simulink model "Lqr_clean"  (R2022a)
settings: Solver=ode3  StartTime=0.0  StopTime=inf  FixedStep=0.005  RelTol=1e-3
undefined symbols (not defined in the file): Angular, Gain, Linear
libraries: robotlib x15
settings Model: Creator=Ronak Jain  LastModifiedBy=Ronak Jain
settings OptimizationCC: EnhancedBackFolding=on  PassReuseOutputArgsAs=Individual arguments  ZeroExternalMemoryAtStartup=off  ZeroInternalMemoryAtStartup=off  MaxStackSize=64  OptimizeBlockOrder=speed  DifferentSizesBufferReuse=on  OptimizationCustomize=off  EfficientTunableParamExpr=on
settings DebuggingCC: ParameterTunabilityLossMsg=error
settings HardwareCC: ProdBitPerPointer=32  ProdBitPerSizeT=32  ProdBitPerPtrDiffT=32  ProdLargestAtomicFloat=None  ProdIntDivRoundTo=Undefined  ProdEndianess=Unspecified  ProdWordSize=32  ProdHWDeviceType=Generic->Unspecified (assume 32-bit Generic)
settings SFSimCC: MATLABDynamicMemAlloc=off
settings RTWCC: SystemTargetFile=ert.tlc  HardwareBoard=Robot Operating System (ROS)  TLCOptions="-aInlineSetEventsForThisBaseRateFcn=TLC_FALSE -aSuppressMultiTaskScheduler=TLC_FALSE  -aRateBasedStepFcn=0"  TemplateMakefile=ert_default_tmf  Toolchain=Catkin  TargetLang=C++
settings CodeAppCC: ForceParamTrailComments=on  IgnoreCustomStorageClasses=off  OperatorAnnotations=on  SimulinkDataObjDesc=on  SFDataObjDesc=on  InsertBlockDesc=on

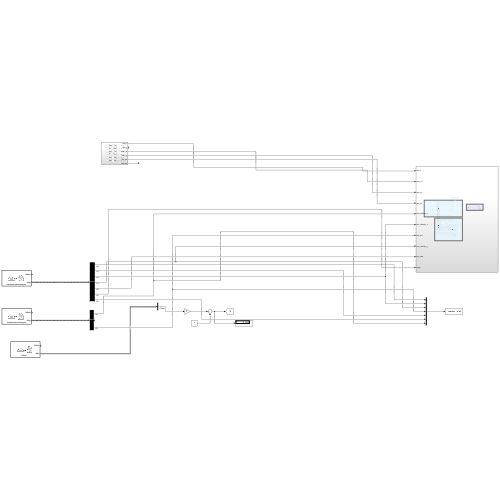
[thumbnail: Simulink's stored preview of the top-level diagram]
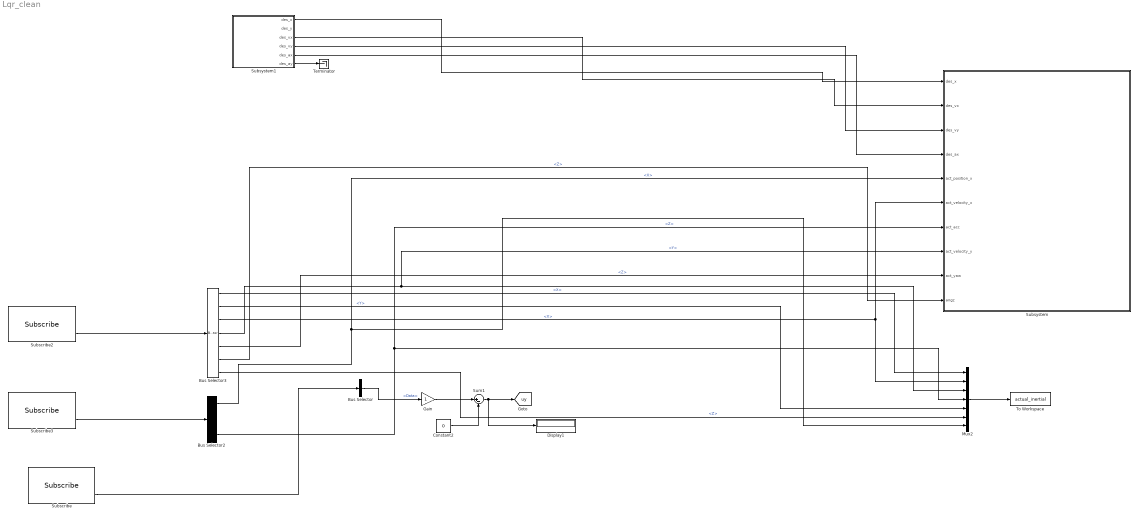
== system Lqr_clean ==
  Bus Selector : BusSelector  OutputSignals=Data
  Bus Selector2 : BusSelector  OutputSignals=LinearAcceleration.X,LinearAcceleration.Y,LinearAcceleration.Z
  Bus Selector3 : BusSelector  OutputSignals=Pose.Pose.Position.X,Pose.Pose.Position.Y,Twist.Twist.Linear.X,Twist.Twist.Linear.Y,Pose.Pose.Orientation.Z,Twist.Twist.Angular.Z,Twist.Twist.Linear.Z
  Constant2 : Constant  Value=0
  Display1 : Display
  Gain : Gain
  Mux2 : Mux  Inputs=7
  Subscribe : robotlib/Subscribe  topicSource=Select from ROS network  topic=/offset  messageType=std_msgs/Float32  SampleTime=-1  legacyBusStruct=off  messageQueueLength=1
  Subscribe2 : robotlib/Subscribe  topicSource=Select from ROS network  topic=/camera/odom/sample  messageType=nav_msgs/Odometry  SampleTime=-1  legacyBusStruct=off  messageQueueLength=1
  Subscribe3 : robotlib/Subscribe  topicSource=Select from ROS network  topic=/camera/accel/sample  messageType=sensor_msgs/Imu  SampleTime=-1  legacyBusStruct=off  messageQueueLength=1
  Subsystem : Subsystem
  Subsystem1 : Subsystem
  Sum1 : Sum  Inputs=|+-
  Terminator : Terminator
  To Workspace : ToWorkspace  VariableName=actual_inertial  SaveFormat=Timeseries  SampleTime=-1
  tag scope: uy=global
  wires:
  Subscribe/2 -> Bus Selector/1
  Bus Selector3/1 -> Mux2/1  "<X>"
  Subsystem1/6(des_ay) -> Terminator/1
  Constant2/1 -> Sum1/2
  Subsystem1/3(des_vx) -> Subsystem/2(des_vx)
  Bus Selector2/1 -> Mux2/7, Subsystem/5(act_position_x)  "<X>"
  Gain/1 -> Sum1/1
  Subscribe3/2 -> Bus Selector2/1
  Subsystem1/5(des_ax) -> Subsystem/4(des_ax)
  Sum1/1 -> Display1/1, [uy]
  Subscribe2/2 -> Bus Selector3/1
  Bus Selector3/7 -> Mux2/6  "<Z>"
  Mux2/1 -> To Workspace/1
  Bus Selector3/3 -> Subsystem/6(act_velocity_x), Mux2/2  "<X>"
  Bus Selector3/5 -> Subsystem/9(act_yaw)  "<Z>"
  Bus Selector/1 -> Gain/1  "<Data>"
  Bus Selector3/4 -> Subsystem/8(act_velocity_y), Mux2/3  "<Y>"
  Bus Selector2/3 -> Subsystem/7(act_acc), Mux2/4  "<Z>"
  Subsystem1/4(des_vy) -> Subsystem/3(des_vy)
  Bus Selector3/6 -> Subsystem/10(angz)  "<Z>"
  Bus Selector3/2 -> Mux2/5  "<Y>"
  Subsystem1/1(des_x) -> Subsystem/1(des_x)

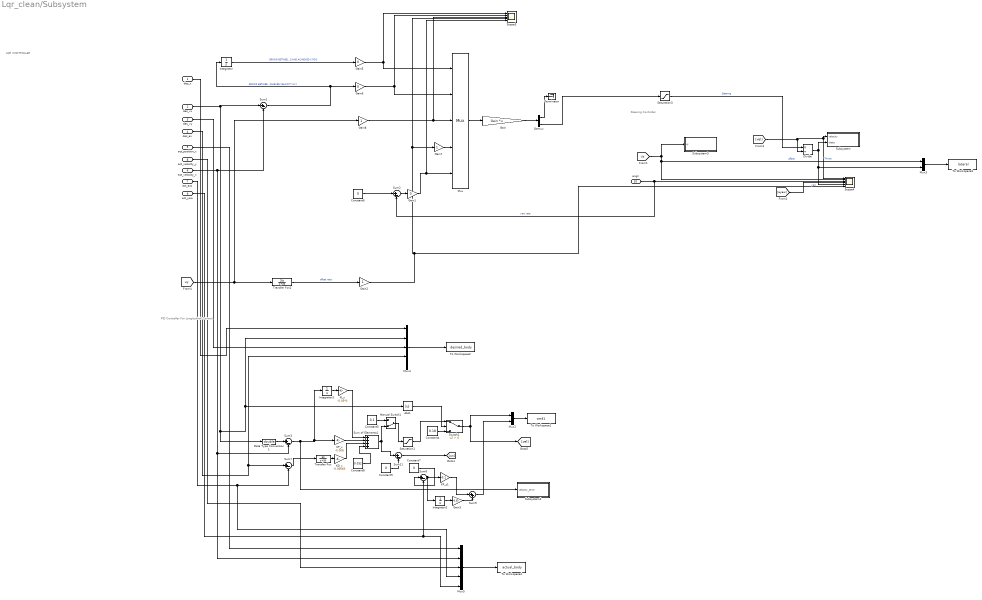
== system Lqr_clean/Subsystem ==
  note: Steering Controller
  note: LQR CONTROLLER
  note: PID Controller
      | For Longitudinal
      | Control.
  des_x : Inport
  des_vx : Inport  Port=2
  des_vy : Inport  Port=3
  des_ax : Inport  Port=4
  act_position_x : Inport  Port=5
  act_velocity_x : Inport  Port=6
  act_acc : Inport  Port=7
  act_velocity_y : Inport  Port=8
  act_yaw : Inport  Port=9
  angz : Inport  Port=10
  Abs1 : Abs  SaturateOnIntegerOverflow=off
  Constant4 : Constant  Value=0.18
  Constant5 : Constant  Value=0.1
  Constant6 : Constant  Value=0
  Constant7 : Constant  Value=0
  Constant8 : Constant  Value=0.032
  Constant9 : Constant  Value=0
  Data Type Conversion1 : DataTypeConversion  OutDataTypeStr=double  SaturateOnIntegerOverflow=off  RndMeth=Floor
  Demux : Demux  Outputs=2
  Divide : Product  Inputs=*/
  Gain : Gain  Gain=Gain  Multiplication=Matrix(K*u)
  Gain1 : Gain  Gain=0
  Gain2 : Gain
  Gain3 : Gain  Gain=-0.33
  Gain5 : Gain  Gain=0
  Gain6 : Gain  Gain=0
  Gain7 : Gain
  Gain8 : Gain
  Integrator : Integrator
  Integrator2 : Integrator
  Integrator3 : Integrator
  KD_x : Gain  Gain=-0.00083
  KI_x : Gain  Gain=-0.05*0
  KP_x : Gain  Gain=-0.008
  KP_z1 : Gain  Gain=-0.1
  Manual Switch1 : ManualSwitch  CurrentSetting=0
  Mux : Mux  Inputs=5
  Mux2 : Mux  Inputs=2
  Mux3 : Mux  Inputs=2
  Mux4 : Mux  Inputs=5
  Mux5 : Mux  Inputs=5
  Saturation1 : Saturate  LowerLimit=-0.2
  Saturation3 : Saturate  UpperLimit=0.7  LowerLimit=-0.7
  Scope3 : Scope  NumInputPorts=5
  Scope4 : Scope  NumInputPorts=6
  Subsystem : Subsystem
  Subsystem2 : Subsystem
  Subsystem3 : Subsystem
  Sum of Elements1 : Sum  Inputs=++++
  Sum{1..3,7..8,11} (6 alike) : Sum  Inputs=|+-
  Sum9 : Sum  Inputs=|++
  Switch1 : Switch  Criteria=u2 > Threshold  SaturateOnIntegerOverflow=off  InputSameDT=off
  Terminator : Terminator
  To Workspace1 : ToWorkspace  VariableName=cmd1  SaveFormat=Timeseries  SampleTime=-1
  To Workspace2 : ToWorkspace  VariableName=desired_body  SaveFormat=Timeseries  SampleTime=-1
  To Workspace3 : ToWorkspace  VariableName=lateral  SaveFormat=Timeseries  SampleTime=-1
  To Workspace4 : ToWorkspace  VariableName=actual_body  SaveFormat=Timeseries  SampleTime=-1
  Transfer Fcn : TransferFcn  Numerator=[50]  Denominator=[1 50]
  Transfer Fcn2 : TransferFcn  Numerator=[20 0]  Denominator=[1 20]
  wires:
  [uy] -> Subsystem3/1(uy), Mux3/1, Scope4/2  "offset"
  angz/1 -> Sum2/2, Scope4/3  "yaw rate"
  [ayaw] -> Scope4/4  "yaw"
  Mux3/1 -> To Workspace3/1
  [vel] -> Subsystem/1(velocity), Scope4/1, Divide/2  "Thrust"
  Sum1/1 -> Integrator/1, Gain6/1  "ERROR BETWEEN DESIRED VELOXITY IN X AND ACHIEVED VELOCITY IN X"
  Integrator/1 -> Gain5/1  "ERROR BETWEEN DESIRED X POS AND ACHIEVED X POS"
  [uy] -> Transfer Fcn2/1, Gain8/1
  Transfer Fcn2/1 -> Gain2/1  "offset rate"
  Sum2/1 -> Gain1/1
  Mux/1 -> Gain/1
  Gain/1 -> Demux/1
  Demux/2 -> Saturation3/1
  Constant6/1 -> Sum2/1
  Saturation3/1 -> Divide/1  "Steering"
  Gain1/1 -> Scope3/5, Mux/5
  Gain2/1 -> Scope4/6, Gain7/1, Scope3/4
  Divide/1 -> Scope4/5, Mux3/2, Subsystem/2(theta)
  des_x/1 -> Mux4/1
  Constant7/1 -> Sum8/1
  Abs1/1 -> Switch1/2
  Constant8/1 -> Sum of Elements1/4
  act_velocity_x/1 -> Sum1/2, Mux5/2, Sum3/2
  des_vy/1 -> Mux4/3
  Sum7/1 -> Transfer Fcn/1
  Transfer Fcn/1 -> KD_x/1
  act_velocity_y/1 -> Mux5/3
  Integrator3/1 -> KI_x/1
  act_yaw/1 -> Mux5/5, Sum8/2
  Gain3/1 -> Sum9/2
  act_acc/1 -> Mux5/4, Sum7/2
  Sum9/1 -> Mux2/2
  Mux2/1 -> To Workspace1/1
  Data Type Conversion1/1 -> Sum3/1
  KP_z1/1 -> Sum9/1
  Mux5/1 -> To Workspace4/1
  Constant9/1 -> Sum11/2
  Constant5/1 -> Manual Switch1/1
  Switch1/1 -> [vel], Mux2/1
  Mux4/1 -> To Workspace2/1
  Sum of Elements1/1 -> Sum11/1, Manual Switch1/2
  act_position_x/1 -> Mux5/1
  des_vx/1 -> Data Type Conversion1/1, Mux4/2, Abs1/1, Sum1/1
  Sum8/1 -> Integrator2/1, KP_z1/1
  des_ax/1 -> Mux4/4, Sum7/1
  KD_x/1 -> Sum of Elements1/3
  Constant4/1 -> Switch1/3
  Saturation1/1 -> Switch1/1
  Integrator2/1 -> Gain3/1
  KP_x/1 -> Sum of Elements1/2
  Sum11/1 -> [ux]
  Sum3/1 -> KP_x/1, Integrator3/1, Subsystem2/1(velocity_error)
  KI_x/1 -> Sum of Elements1/1
  Manual Switch1/1 -> Saturation1/1
  Gain5/1 -> Mux/1, Scope3/1
  Gain6/1 -> Mux/2, Scope3/2
  Gain7/1 -> Mux/4
  Gain8/1 -> Scope3/3, Mux/3
  Demux/1 -> Terminator/1

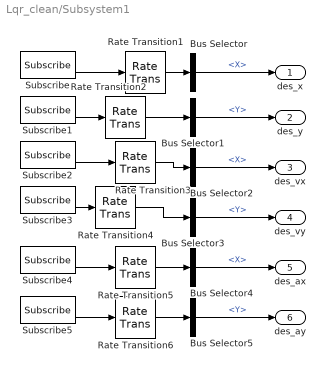
== system Lqr_clean/Subsystem1 ==
  Bus Selector : BusSelector  OutputSignals=Position.X
  Bus Selector1 : BusSelector  OutputSignals=Position.Y
  Bus Selector2 : BusSelector  OutputSignals=Linear.X
  Bus Selector3 : BusSelector  OutputSignals=Linear.Y
  Bus Selector4 : BusSelector  OutputSignals=Linear.X
  Bus Selector5 : BusSelector  OutputSignals=Linear.Y
  Rate Transition{1..6} (6 alike) : RateTransition
  Subscribe : robotlib/Subscribe  topicSource=Select from ROS network  topic=/des_x  messageType=geometry_msgs/Pose  SampleTime=-1  legacyBusStruct=off  messageQueueLength=1
  Subscribe1 : robotlib/Subscribe  topicSource=Select from ROS network  topic=/des_y  messageType=geometry_msgs/Pose  SampleTime=-1  legacyBusStruct=off  messageQueueLength=1
  Subscribe2 : robotlib/Subscribe  topicSource=Select from ROS network  topic=/des_vx  messageType=geometry_msgs/Twist  SampleTime=-1  legacyBusStruct=off  messageQueueLength=1
  Subscribe3 : robotlib/Subscribe  topicSource=Select from ROS network  topic=/des_vy  messageType=geometry_msgs/Twist  SampleTime=-1  legacyBusStruct=off  messageQueueLength=1
  Subscribe4 : robotlib/Subscribe  topicSource=Select from ROS network  topic=/des_ax  messageType=geometry_msgs/Accel  SampleTime=-1  legacyBusStruct=off  messageQueueLength=1
  Subscribe5 : robotlib/Subscribe  topicSource=Select from ROS network  topic=/des_ay  messageType=geometry_msgs/Accel  SampleTime=-1  legacyBusStruct=off  messageQueueLength=1
  des_x : Outport
  des_y : Outport  Port=2
  des_vx : Outport  Port=3
  des_vy : Outport  Port=4
  des_ax : Outport  Port=5
  des_ay : Outport  Port=6
  wires:
  Subscribe1/2 -> Rate Transition2/1
  Bus Selector1/1 -> des_y/1  "<Y>"
  Bus Selector3/1 -> des_vy/1  "<Y>"
  Subscribe/2 -> Rate Transition1/1
  Bus Selector/1 -> des_x/1  "<X>"
  Bus Selector2/1 -> des_vx/1  "<X>"
  Bus Selector4/1 -> des_ax/1  "<X>"
  Bus Selector5/1 -> des_ay/1  "<Y>"
  Rate Transition1/1 -> Bus Selector/1
  Rate Transition2/1 -> Bus Selector1/1
  Subscribe2/2 -> Rate Transition3/1
  Rate Transition3/1 -> Bus Selector2/1
  Subscribe3/2 -> Rate Transition4/1
  Rate Transition4/1 -> Bus Selector3/1
  Subscribe4/2 -> Rate Transition5/1
  Rate Transition5/1 -> Bus Selector4/1
  Subscribe5/2 -> Rate Transition6/1
  Rate Transition6/1 -> Bus Selector5/1

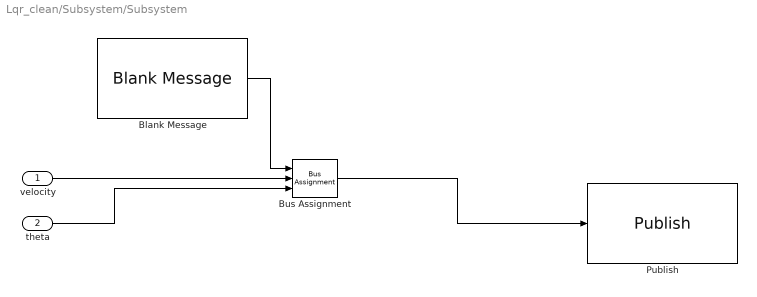
== system Lqr_clean/Subsystem/Subsystem ==
  velocity : Inport
  theta : Inport  Port=2
  Blank Message : robotlib/Blank Message  messageClass=Message  entityType=geometry_msgs/Twist  messageType=geometry_msgs/Twist  SampleTime=-1  legacyBusStruct=off
  Bus Assignment : BusAssignment  AssignedSignals=Linear.X,Angular.Z
  Publish : robotlib/Publish  topicSource=Specify your own  topic=/move_velocity  messageType=geometry_msgs/Twist  legacyBusStruct=off  messageQueueLength=1
  wires:
  theta/1 -> Bus Assignment/3
  Blank Message/1 -> Bus Assignment/1
  velocity/1 -> Bus Assignment/2
  Bus Assignment/1 -> Publish/1

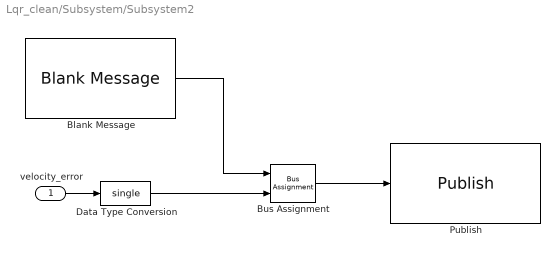
== system Lqr_clean/Subsystem/Subsystem2 ==
  velocity_error : Inport
  Blank Message : robotlib/Blank Message  messageClass=Message  entityType=std_msgs/Float32  messageType=std_msgs/Float32  SampleTime=-1  legacyBusStruct=off
  Bus Assignment : BusAssignment  AssignedSignals=Data
  Data Type Conversion : DataTypeConversion  OutDataTypeStr=single  SaturateOnIntegerOverflow=off  RndMeth=Floor
  Publish : robotlib/Publish  topicSource=Specify your own  topic=/vel_error  messageType=std_msgs/Float32  legacyBusStruct=off  messageQueueLength=1
  wires:
  Blank Message/1 -> Bus Assignment/1
  Bus Assignment/1 -> Publish/1
  velocity_error/1 -> Data Type Conversion/1
  Data Type Conversion/1 -> Bus Assignment/2

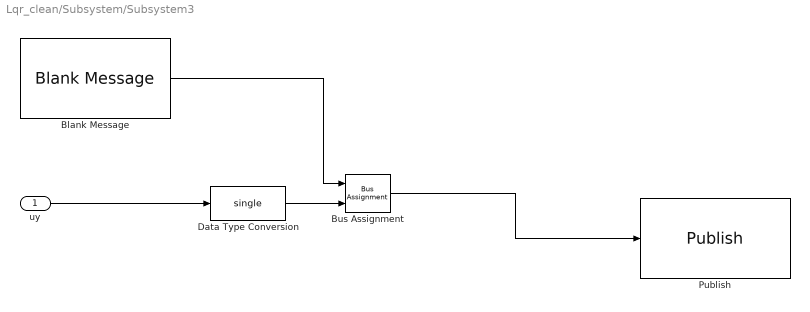
== system Lqr_clean/Subsystem/Subsystem3 ==
  uy : Inport
  Blank Message : robotlib/Blank Message  messageClass=Message  entityType=std_msgs/Float32  messageType=std_msgs/Float32  SampleTime=-1  legacyBusStruct=off
  Bus Assignment : BusAssignment  AssignedSignals=Data
  Data Type Conversion : DataTypeConversion  OutDataTypeStr=single  SaturateOnIntegerOverflow=off  RndMeth=Floor
  Publish : robotlib/Publish  topicSource=Specify your own  topic=/uy  messageType=std_msgs/Float32  legacyBusStruct=off  messageQueueLength=1
  wires:
  uy/1 -> Data Type Conversion/1
  Data Type Conversion/1 -> Bus Assignment/2
  Blank Message/1 -> Bus Assignment/1
  Bus Assignment/1 -> Publish/1
